simulink model "OilP_VD"  (R2016b)
settings: configuration reference "CodeGenConfigSet" (kept outside this file)
values from neighbouring files (symbols this model uses):
  Oil_facPT1FltP_C = Calibration.Parameter    [init_OilP_VD.m]    (also in init_OilP_VD_SIL.m = Simulink.Parameter)
  Oil_pTransStgDfl_C = Calibration.Parameter    [init_OilP_VD.m]    (also in init_OilP_VD_SIL.m = Simulink.Parameter)
  Oil_RmpSlpPNeg_C = Calibration.Parameter    [init_OilP_VD.m]    (also in init_OilP_VD_SIL.m = Simulink.Parameter)
  Oil_RmpSlpPPos_C = Calibration.Parameter    [init_OilP_VD.m]    (also in init_OilP_VD_SIL.m = Simulink.Parameter)
  Oil_swtPresSensTyp_C = Calibration.Parameter    [init_OilP_VD.m]    (also in init_OilP_VD_SIL.m = Simulink.Parameter)
  SigTst_pOilPSwmp_C = Calibration.Parameter    [init_OilP_VD.m]    (also in init_OilP_VD_SIL.m = Simulink.Parameter)
  SigTst_swtOilPSwmp_C = Calibration.Parameter    [init_OilP_VD.m]    (also in init_OilP_VD_SIL.m = Simulink.Parameter)
undefined symbols (not defined in the file or in its folder): CEngDst_switch_conv, OilP_VD_DT, Switch_conv
libraries: CXLib x4
settings Model: Creator=Wollf  LastModifiedBy=xinchangran
settings ConfigSetRef: SourceLocation=Base Workspace

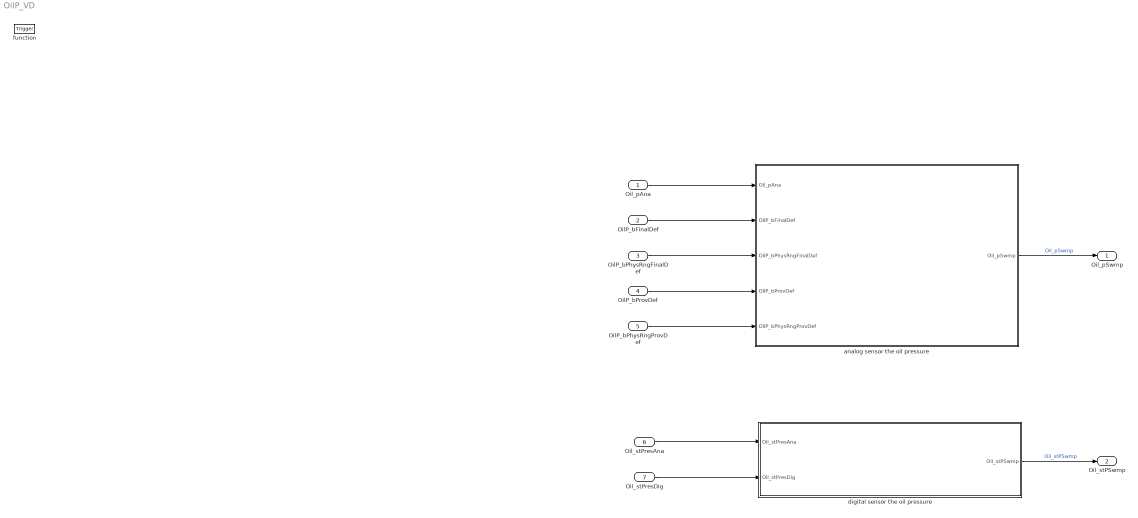
== system OilP_VD ==
  Oil_pAna : Inport  Tag=kPa  Description=Oil pressure for analog input  OutMin=0  OutMax=1200  OutDataTypeStr=AirPressure_kPa
  OilP_bFinalDef : Inport  Description=Status sensor of the oil pressure finally defect  Port=2  OutMin=0  OutMax=1  OutDataTypeStr=boolean
  OilP_bPhysRngFinalDef : Inport  Description=Status sensor of the oil pressure physical signal range check finally defect  Port=3  OutMin=0  OutMax=1  OutDataTypeStr=boolean
  OilP_bProvDef : Inport  Description=Status sensor of the oil pressure temporary defect  Port=4  OutMin=0  OutMax=1  OutDataTypeStr=boolean
  OilP_bPhysRngProvDef : Inport  Description=Status sensor of the oil pressure physical signal range check temporary defect  Port=5  OutMin=0  OutMax=1  OutDataTypeStr=boolean
  Oil_stPresAna : Inport  Description=Oil pressure status for analog input  Port=6  OutMin=0  OutMax=1  OutDataTypeStr=boolean
  Oil_stPresDig : Inport  Description=Oil pressure status for digital input  Port=7  OutMin=0  OutMax=1  OutDataTypeStr=boolean
  function : TriggerPort  TriggerType=function-call  VariantControl=Variant
  analog sensor the oil pressure : Subsystem
  digital sensor the oil pressure : Subsystem
  Oil_pSwmp : Outport  Tag=kPa  Description=Filtered oil pressure value  OutMin=0  OutMax=1200  OutDataTypeStr=AirPressure_kPa
  Oil_stPSwmp : Outport  Description=sensor out oil pressure status  Port=2  OutMin=0  OutMax=1  OutDataTypeStr=boolean
  wires:
  Oil_pAna/1 -> analog sensor the oil pressure/1(Oil_pAna)
  OilP_bFinalDef/1 -> analog sensor the oil pressure/2(OilP_bFinalDef)
  OilP_bPhysRngFinalDef/1 -> analog sensor the oil pressure/3(OilP_bPhysRngFinalDef)
  OilP_bProvDef/1 -> analog sensor the oil pressure/4(OilP_bProvDef)
  OilP_bPhysRngProvDef/1 -> analog sensor the oil pressure/5(OilP_bPhysRngProvDef)
  analog sensor the oil pressure/1(Oil_pSwmp) -> Oil_pSwmp/1  "Oil_pSwmp"
  Oil_stPresAna/1 -> digital sensor the oil pressure/1(Oil_stPresAna)
  Oil_stPresDig/1 -> digital sensor the oil pressure/2(Oil_stPresDig)
  digital sensor the oil pressure/1(Oil_stPSwmp) -> Oil_stPSwmp/1  "Oil_stPSwmp"

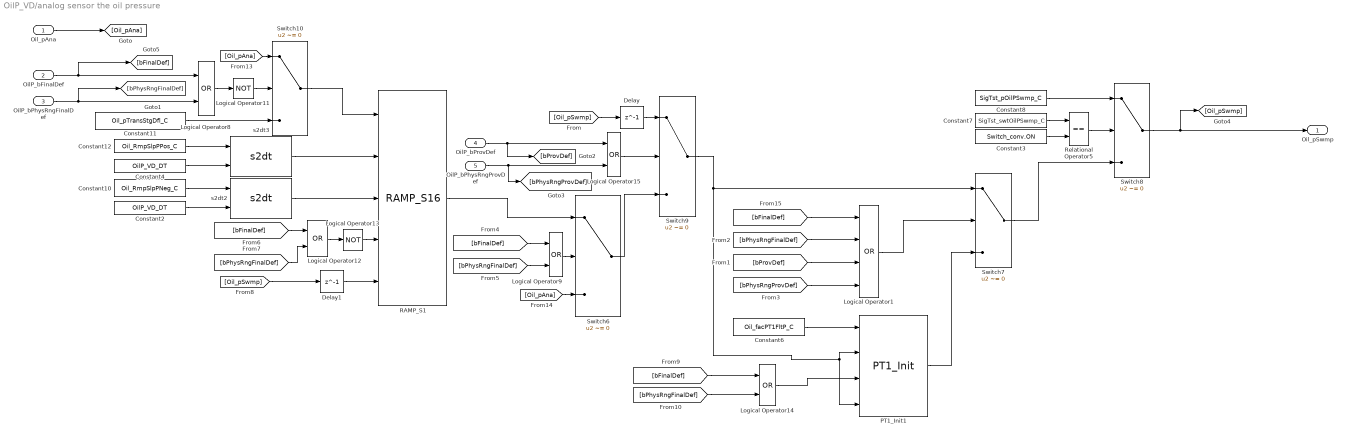
== system OilP_VD/analog sensor the oil pressure ==
  Oil_pAna : Inport  Tag=kPa  Description=Oil pressure for analog input  OutMin=0  OutMax=1200  OutDataTypeStr=AirPressure_kPa
  OilP_bFinalDef : Inport  Description=Status sensor of the oil pressure finally defect  Port=2  OutMin=0  OutMax=1  OutDataTypeStr=boolean
  OilP_bPhysRngFinalDef : Inport  Description=Status sensor of the oil pressure physical signal range check finally defect  Port=3  OutMin=0  OutMax=1  OutDataTypeStr=boolean
  OilP_bProvDef : Inport  Description=Status sensor of the oil pressure temporary defect  Port=4  OutMin=0  OutMax=1  OutDataTypeStr=boolean
  OilP_bPhysRngProvDef : Inport  Description=Status sensor of the oil pressure physical signal range check temporary defect  Port=5  OutMin=0  OutMax=1  OutDataTypeStr=boolean
  Constant10 : Constant  Value=Oil_RmpSlpPNeg_C  SampleTime=-1
  Constant11 : Constant  Value=Oil_pTransStgDfl_C  SampleTime=-1
  Constant12 : Constant  Value=Oil_RmpSlpPPos_C  SampleTime=-1
  Constant2 : Constant  Value=OilP_VD_DT  OutDataTypeStr=int16  SampleTime=-1
  Constant3 : Constant  Value=Switch_conv.ON  OutDataTypeStr=Inherit: Inherit via back propagation
  Constant4 : Constant  Value=OilP_VD_DT  OutDataTypeStr=int16  SampleTime=-1
  Constant6 : Constant  Value=Oil_facPT1FltP_C  SampleTime=-1
  Constant7 : Constant  Value=SigTst_swtOilPSwmp_C  SampleTime=-1
  Constant8 : Constant  Value=SigTst_pOilPSwmp_C  SampleTime=-1
  Delay : Delay  DialogController=Simulink.DDGSource  DelayLength=1  InitialCondition=0
  Delay1 : Delay  DialogController=Simulink.DDGSource  DelayLength=1  InitialCondition=0
  Logical Operator1 : Logic  Operator=OR  Inputs=4  OutDataTypeStr=boolean
  Logical Operator11 : Logic  Operator=NOT  AllPortsSameDT=off  OutDataTypeStr=boolean
  Logical Operator{8..9,12,14..15} (5 alike) : Logic  Operator=OR  OutDataTypeStr=boolean
  Logical Operator13 : Logic  Operator=NOT  AllPortsSameDT=off  OutDataTypeStr=boolean
  PT1_Init1 : CXLib/PT1_Init
  RAMP_S1 : CXLib/RAMP_S16
  Relational Operator5 : RelationalOperator  Operator===  OutDataTypeStr=boolean  RndMeth=Simplest  InputSameDT=on
  Switch{6..7,9..10} (4 alike) : Switch  Criteria=u2 ~= 0  InputSameDT=on
  Switch8 : Switch  Criteria=u2 ~= 0  Threshold=CEngDst_switch_conv.OFF  InputSameDT=on
  s2dt2 : CXLib/s2dt
  s2dt3 : CXLib/s2dt
  Oil_pSwmp : Outport
  wires:
  [bFinalDef] -> Logical Operator1/1
  OilP_bFinalDef/1 -> [bFinalDef], Logical Operator8/1
  [bPhysRngFinalDef] -> Logical Operator9/2
  Switch7/1 -> Switch8/3
  Oil_pAna/1 -> [Oil_pAna]
  Switch6/1 -> Switch9/3
  Switch8/1 -> Oil_pSwmp/1, [Oil_pSwmp]
  Logical Operator1/1 -> Switch7/2
  Logical Operator11/1 -> Switch10/2
  Logical Operator15/1 -> Switch9/2
  RAMP_S1/1 -> Switch6/1
  OilP_bProvDef/1 -> [bProvDef], Logical Operator15/1
  Constant11/1 -> Switch10/3
  [bProvDef] -> Logical Operator1/3
  OilP_bPhysRngProvDef/1 -> [bPhysRngProvDef], Logical Operator15/2
  s2dt2/1 -> RAMP_S1/3
  PT1_Init1/1 -> Switch7/3
  Switch10/1 -> RAMP_S1/1
  Logical Operator8/1 -> Logical Operator11/1
  Logical Operator12/1 -> Logical Operator13/1
  OilP_bPhysRngFinalDef/1 -> [bPhysRngFinalDef], Logical Operator8/2
  Constant6/1 -> PT1_Init1/1
  [bPhysRngFinalDef] -> Logical Operator1/2
  Logical Operator9/1 -> Switch6/2
  s2dt3/1 -> RAMP_S1/2
  [bPhysRngProvDef] -> Logical Operator1/4
  Constant7/1 -> Relational Operator5/1
  Switch9/1 -> PT1_Init1/2, PT1_Init1/4, Switch7/1
  Constant8/1 -> Switch8/1
  Constant3/1 -> Relational Operator5/2
  [bFinalDef] -> Logical Operator9/1
  Relational Operator5/1 -> Switch8/2
  [bFinalDef] -> Logical Operator12/1
  Delay1/1 -> RAMP_S1/5
  Constant4/1 -> s2dt3/2
  [Oil_pSwmp] -> Delay/1
  [Oil_pAna] -> Switch10/1
  [bPhysRngFinalDef] -> Logical Operator14/2
  [bPhysRngFinalDef] -> Logical Operator12/2
  Logical Operator14/1 -> PT1_Init1/3
  Constant2/1 -> s2dt2/2
  [Oil_pSwmp] -> Delay1/1
  Logical Operator13/1 -> RAMP_S1/4
  [Oil_pAna] -> Switch6/3
  Delay/1 -> Switch9/1
  Constant12/1 -> s2dt3/1
  [bFinalDef] -> Logical Operator14/1
  Constant10/1 -> s2dt2/1

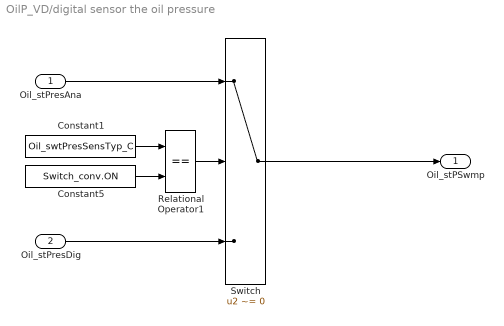
== system OilP_VD/digital sensor the oil pressure ==
  Oil_stPresAna : Inport  Description=Oil pressure status for analog input  OutMin=0  OutMax=1  OutDataTypeStr=boolean
  Oil_stPresDig : Inport  Description=Oil pressure status for digital input  Port=2  OutMin=0  OutMax=1  OutDataTypeStr=boolean
  Constant1 : Constant  Value=Oil_swtPresSensTyp_C  SampleTime=-1
  Constant5 : Constant  Value=Switch_conv.ON  OutDataTypeStr=Inherit: Inherit via back propagation
  Relational Operator1 : RelationalOperator  Operator===  OutDataTypeStr=boolean  RndMeth=Simplest  InputSameDT=on
  Switch : Switch  Criteria=u2 ~= 0  InputSameDT=on
  Oil_stPSwmp : Outport  Description=sensor out oil pressure status  OutMin=0  OutMax=1  OutDataTypeStr=boolean
  wires:
  Oil_stPresAna/1 -> Switch/1
  Oil_stPresDig/1 -> Switch/3
  Constant5/1 -> Relational Operator1/2
  Constant1/1 -> Relational Operator1/1
  Relational Operator1/1 -> Switch/2
  Switch/1 -> Oil_stPSwmp/1
